simulink model "Sistema_Final"  (R2023a)
settings: Solver=VariableStepAuto  StartTime=0.0  StopTime=30  MaxStep=0.001  RelTol=1e-3
libraries: slpidlib x1
settings Model: Creator=sally  LastModifiedBy=ALEXANDER TORRES
settings DataIOCC: ReturnWorkspaceOutputs=off  TimeSaveName=t
settings DebuggingCC: AlgebraicLoopMsg=none

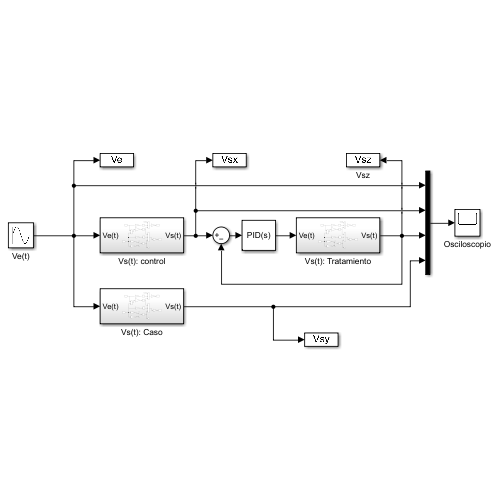
[thumbnail: Simulink's stored preview of the top-level diagram]
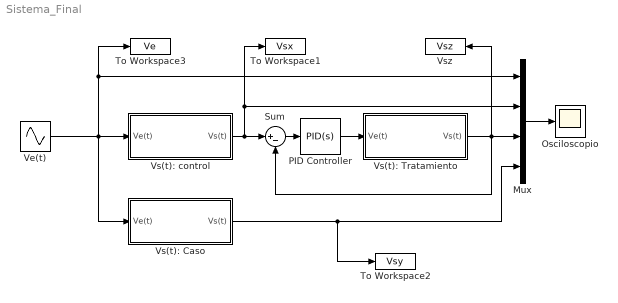
== system Sistema_Final ==
  Mux : Mux
  Osciloscopio : Scope
  PID Controller : slpidlib/PID Controller  Controller=PID  Form=Parallel  TimeDomain=Continuous-time  UseExternalTs=off  SampleTime=-1  IntegratorMethod=Forward Euler  FilterMethod=Forward Euler  ControllerParametersSource=internal  P=30.7048930701238  I=215.144071879233  UseKiTs=off  D=0.336288499629592  N=47.3374611492195  UseFilter=on  TunerSelectOption=Transfer Function Based (PID Tuner App)  InitialConditionSource=internal  InitialConditionForIntegrator=0  InitialConditionForFilter=0  DifferentiatorICPrevScaledInput=0  ExternalReset=none  TrackingMode=off  Kt=1  LimitOutput=off  SatLimitsSource=internal  UpperSaturationLimit=inf  LowerSaturationLimit=-inf  LinearizeAsGain=on  AntiWindupMode=none  Kb=1  LimitIntegrator=off  UpperIntegratorSaturationLimit=inf  LowerIntegratorSaturationLimit=-inf  POutMin=[]  POutMax=[]  IOutMin=[]  IOutMax=[]  DOutMin=[]  DOutMax=[]  NOutMin=[]  NOutMax=[]  SumOutMin=[]  SumOutMax=[]  SaturationOutMin=[]  SaturationOutMax=[]  PParamMin=[]  PParamMax=[]  IParamMin=[]  IParamMax=[]  DParamMin=[]  DParamMax=[]  NParamMin=[]  NParamMax=[]  KbParamMin=[]  KbParamMax=[]  KtParamMin=[]  KtParamMax=[]  KbOutMin=[]  KbOutMax=[]  KtOutMin=[]  KtOutMax=[]  IntegratorOutMin=[]  IntegratorOutMax=[]  FilterOutMin=[]  FilterOutMax=[]  SumI1OutMin=[]  SumI1OutMax=[]  SumI2OutMin=[]  SumI2OutMax=[]  SumI3OutMin=[]  SumI3OutMax=[]  SumI4OutMin=[]  SumI4OutMax=[]  SumDOutMin=[]  SumDOutMax=[]  DifferentiatorOutMin=[]  DifferentiatorOutMax=[]  FilterDiffOutCoefMin=[]  FilterDiffOutCoefMax=[]  ReciprocalOutMin=[]  ReciprocalOutMax=[]  SumDenOutMin=[]  SumDenOutMax=[]  SumNumOutMin=[]  SumNumOutMax=[]  DivideOutMin=[]  DivideOutMax=[]  UdiffTsProdOutMin=[]  UdiffTsProdOutMax=[]  NTsProdOutMin=[]  NTsProdOutMax=[]  UintegralTsProdOutMin=[]  UintegralTsProdOutMax=[]  UngainTsProdOutMin=[]  UngainTsProdOutMax=[]  ClampingZeroOutDataTypeStr=Inherit: Inherit via back propagation  ClampingZeroOutMin=[]  ClampingZeroOutMax=[]  FilterDenConstantOutDataTypeStr=Inherit: Inherit via back propagation  FilterDenConstantOutMin=[]  FilterDenConstantOutMax=[]  PCopyOutDataTypeStr=Inherit: Inherit via back propagation  PCopyOutMin=[]  PCopyOutMax=[]  NCopyOutDataTypeStr=Inherit: Inherit via back propagation  NCopyOutMin=[]  NCopyOutMax=[]  IntegratorContinuousStateAttributes=''  IntegratorStateMustResolveToSignalObject=off  IntegratorRTWStateStorageClass=Auto  FilterContinuousStateAttributes=''  FilterStateMustResolveToSignalObject=off  FilterRTWStateStorageClass=Auto  ParallelPVariant=InternalParameters  IdealPVariant=Disabled  IVariant=InternalParameters  DVariant=InternalParameters  IntegratorVariant=Continuous  SatVariant=Disabled  AWVariant=Passthrough  PCopyVariant=Disabled  TRVariant=Disabled  FdbkBlocksVariant=Forward  IdealPFdbkVariant=Disabled  SatFdbkVariant=Disabled  DerivativeFilterVariant=ContFilter  NVariant=InternalParameters  NCopyVariant=Disabled  FilterICVariant=InternalICsFilter  IntegratorICVariant=InternalICs  ExternalResetVariant=Disabled  TRSumVariant=Passthrough  SumFdbkVariant=Disabled  SumVariant=Sum_PID  TsampFilterVariant=InternalTs  TsampNgainVariant=Passthrough  TsampIntegralVariant=Disabled_SignalSpec  ExternalSaturationOutDataTypeStr=Inherit: Same as second input
  Sum : Sum  Inputs=|+-
  To Workspace1 : ToWorkspace  VariableName=Vsx  SampleTime=-1
  To Workspace2 : ToWorkspace  VariableName=Vsy  SampleTime=-1
  To Workspace3 : ToWorkspace  VariableName=Ve  SampleTime=-1
  Ve(t) : Sin  Amplitude=1.5  Frequency=pi  SampleTime=0
  Vs(t): Caso : Subsystem
  Vs(t): Tratamiento : Subsystem
  Vs(t): control : Subsystem
  Vsz : ToWorkspace  VariableName=Vsz  SampleTime=-1
      settings: Tag=Ve
  wires:
  PID Controller/1 -> Vs(t): Tratamiento/1(Ve(t))
  Mux/1 -> Osciloscopio/1
  Sum/1 -> PID Controller/1
  Ve(t)/1 -> To Workspace3/1, Mux/1, Vs(t): control/1(Ve(t)), Vs(t): Caso/1(Ve(t))
  Vs(t): control/1(Vs(t)) -> To Workspace1/1, Mux/2, Sum/1
  Vs(t): Tratamiento/1(Vs(t)) -> Sum/2, Vsz/1, Mux/3
  Vs(t): Caso/1(Vs(t)) -> Mux/4, To Workspace2/1

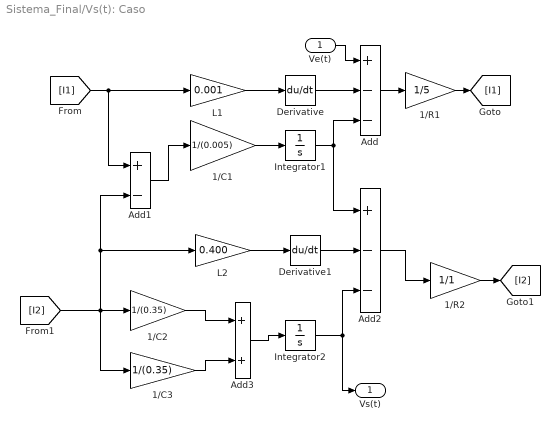
== system Sistema_Final/Vs(t): Caso ==
  Ve(t) : Inport
  1/C1 : Gain  Gain=1/(0.005)
  1/C2 : Gain  Gain=1/(0.35)
  1/C3 : Gain  Gain=1/(0.35)
  1/R1 : Gain  Gain=1/5
  1/R2 : Gain  Gain=1/1
  Add : Sum  Inputs=+--
  Add1 : Sum  Inputs=+-
  Add2 : Sum  Inputs=+--
  Add3 : Sum
  Derivative : Derivative
  Derivative1 : Derivative
  Integrator1 : Integrator
  Integrator2 : Integrator
  L1 : Gain  Gain=0.001
  L2 : Gain  Gain=0.400
  Vs(t) : Outport
  wires:
  1/R2/1 -> [I2]
  Add3/1 -> Integrator2/1
  Add2/1 -> 1/R2/1
  Integrator2/1 -> Add2/3, Vs(t)/1
  1/C3/1 -> Add3/2
  1/R1/1 -> [I1]
  Add1/1 -> 1/C1/1
  Derivative/1 -> Add/2
  Integrator1/1 -> Add/3, Add2/1
  1/C1/1 -> Integrator1/1
  L2/1 -> Derivative1/1
  Add/1 -> 1/R1/1
  1/C2/1 -> Add3/1
  [I1] -> Add1/1, L1/1
  Derivative1/1 -> Add2/2
  Ve(t)/1 -> Add/1
  L1/1 -> Derivative/1
  [I2] -> 1/C3/1, 1/C2/1, L2/1, Add1/2

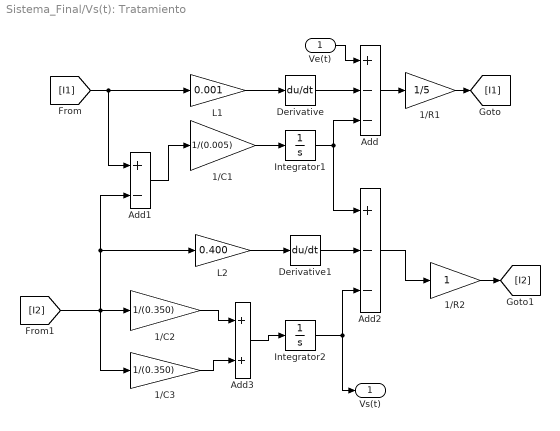
== system Sistema_Final/Vs(t): Tratamiento ==
  Ve(t) : Inport
  1/C1 : Gain  Gain=1/(0.005)
  1/C2 : Gain  Gain=1/(0.350)
  1/C3 : Gain  Gain=1/(0.350)
  1/R1 : Gain  Gain=1/5
  1/R2 : Gain
  Add : Sum  Inputs=+--
  Add1 : Sum  Inputs=+-
  Add2 : Sum  Inputs=+--
  Add3 : Sum
  Derivative : Derivative
  Derivative1 : Derivative
  Integrator1 : Integrator
  Integrator2 : Integrator
  L1 : Gain  Gain=0.001
  L2 : Gain  Gain=0.400
  Vs(t) : Outport
  wires:
  1/R2/1 -> [I2]
  Add3/1 -> Integrator2/1
  Add2/1 -> 1/R2/1
  Integrator2/1 -> Add2/3, Vs(t)/1
  1/C3/1 -> Add3/2
  1/R1/1 -> [I1]
  Add1/1 -> 1/C1/1
  Derivative/1 -> Add/2
  Integrator1/1 -> Add/3, Add2/1
  1/C1/1 -> Integrator1/1
  L2/1 -> Derivative1/1
  Add/1 -> 1/R1/1
  1/C2/1 -> Add3/1
  [I1] -> Add1/1, L1/1
  Derivative1/1 -> Add2/2
  Ve(t)/1 -> Add/1
  L1/1 -> Derivative/1
  [I2] -> 1/C3/1, 1/C2/1, L2/1, Add1/2

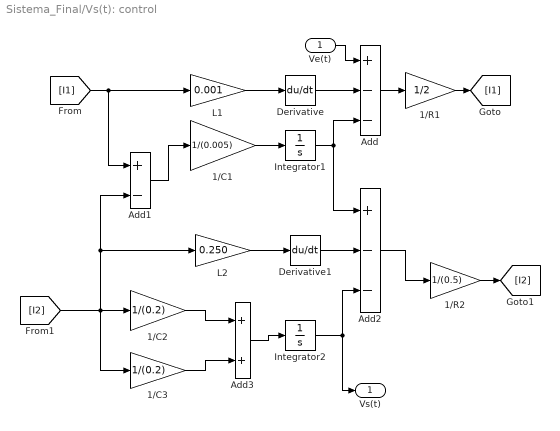
== system Sistema_Final/Vs(t): control ==
  Ve(t) : Inport
  1/C1 : Gain  Gain=1/(0.005)
  1/C2 : Gain  Gain=1/(0.2)
  1/C3 : Gain  Gain=1/(0.2)
  1/R1 : Gain  Gain=1/2
  1/R2 : Gain  Gain=1/(0.5)
  Add : Sum  Inputs=+--
  Add1 : Sum  Inputs=+-
  Add2 : Sum  Inputs=+--
  Add3 : Sum
  Derivative : Derivative
  Derivative1 : Derivative
  Integrator1 : Integrator
  Integrator2 : Integrator
  L1 : Gain  Gain=0.001
  L2 : Gain  Gain=0.250
  Vs(t) : Outport
  wires:
  Ve(t)/1 -> Add/1
  Add1/1 -> 1/C1/1
  1/C1/1 -> Integrator1/1
  Derivative/1 -> Add/2
  L1/1 -> Derivative/1
  Add/1 -> 1/R1/1
  Integrator1/1 -> Add/3, Add2/1
  Integrator2/1 -> Add2/3, Vs(t)/1
  Add2/1 -> 1/R2/1
  Add3/1 -> Integrator2/1
  1/C2/1 -> Add3/1
  1/C3/1 -> Add3/2
  1/R1/1 -> [I1]
  1/R2/1 -> [I2]
  [I1] -> Add1/1, L1/1
  [I2] -> 1/C3/1, 1/C2/1, L2/1, Add1/2
  L2/1 -> Derivative1/1
  Derivative1/1 -> Add2/2
